simulink model "lab3"  (R2020a)
settings: Solver=VariableStepAuto  StartTime=0.0  StopTime=0.5  RelTol=1e-3
values from neighbouring files (symbols this model uses):
  Bx = 0.0094    [controller_design.m]
  By = 0.0091    [controller_design.m]
  Jex = 4.36*10^(-4)    (= 0.000436)    [controller_design.m]
  Jey = 3*10^(-4)    (= 0.0003)    [controller_design.m]
  Kax = 1    [controller_design.m]
  Kay = 1    [controller_design.m]
  Ktx = 0.49    [controller_design.m]
  Kty = 0.49    [controller_design.m]
  s = tf("s")    [controller_design.m]    (also in getLL.m; getLLI.m)
  Ts = 0.0001    [controller_design.m]
libraries: cstblocks x4, simulink x1
settings Model: Creator=brucecui  LastModifiedBy=brucecui

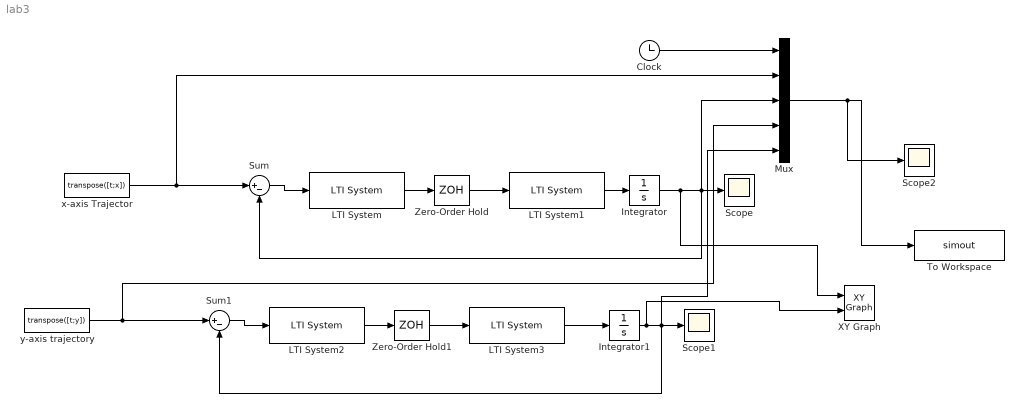
== system lab3 ==
  Clock : Clock
  Integrator : Integrator
  Integrator1 : Integrator
  LTI System : cstblocks/LTI System  sys=LLIlowBandWidthXD  IC=[]
  LTI System1 : cstblocks/LTI System  sys=Kax*Ktx*1/(Jex*s+Bx)  IC=[]
  LTI System2 : cstblocks/LTI System  sys=LLIlowBandWidthYD  IC=[]
  LTI System3 : cstblocks/LTI System  sys=Kay*Kty*1/(Jey*s+By)  IC=[]
  Mux : Mux  Inputs=5
  Scope : Scope
  Scope1 : Scope
  Scope2 : Scope
  Sum : Sum  Inputs=|+-
  Sum1 : Sum  Inputs=|+-
  To Workspace : ToWorkspace  VariableName=simout  SaveFormat=Timeseries  SampleTime=-1
  XY Graph : simulink/Sinks/XY Graph  xmin=-1  xmax=1  ymin=-1  ymax=1  st=-1
  Zero-Order Hold : ZeroOrderHold  SampleTime=Ts
  Zero-Order Hold1 : ZeroOrderHold  SampleTime=Ts
  x-axis Trajector : FromWorkspace  VariableName=transpose([t;x])  SampleTime=Ts
  y-axis trajectory : FromWorkspace  VariableName=transpose([t;y])  SampleTime=Ts
  wires:
  LTI System/1 -> Zero-Order Hold/1
  Zero-Order Hold/1 -> LTI System1/1
  Sum/1 -> LTI System/1
  x-axis Trajector/1 -> Mux/2, Sum/1
  LTI System1/1 -> Integrator/1
  Integrator/1 -> XY Graph/1, Mux/3, Sum/2, Scope/1
  Clock/1 -> Mux/1
  Integrator1/1 -> XY Graph/2, Sum1/2, Mux/5, Scope1/1
  LTI System3/1 -> Integrator1/1
  LTI System2/1 -> Zero-Order Hold1/1
  y-axis trajectory/1 -> Mux/4, Sum1/1
  Sum1/1 -> LTI System2/1
  Zero-Order Hold1/1 -> LTI System3/1
  Mux/1 -> To Workspace/1, Scope2/1
